simulink model "Closed_loop_Model_P_Controller"  (R2024b)
settings: Solver=VariableStepAuto  StartTime=0.0  StopTime=10.0  RelTol=1e-3
settings Model: Creator=Zohaib  LastModifiedBy=Zohaib

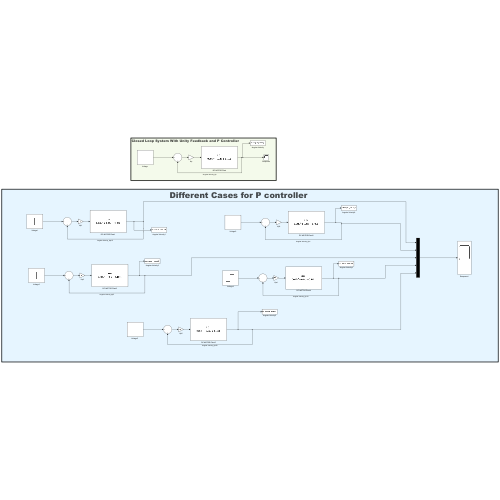
[thumbnail: Simulink's stored preview of the top-level diagram]
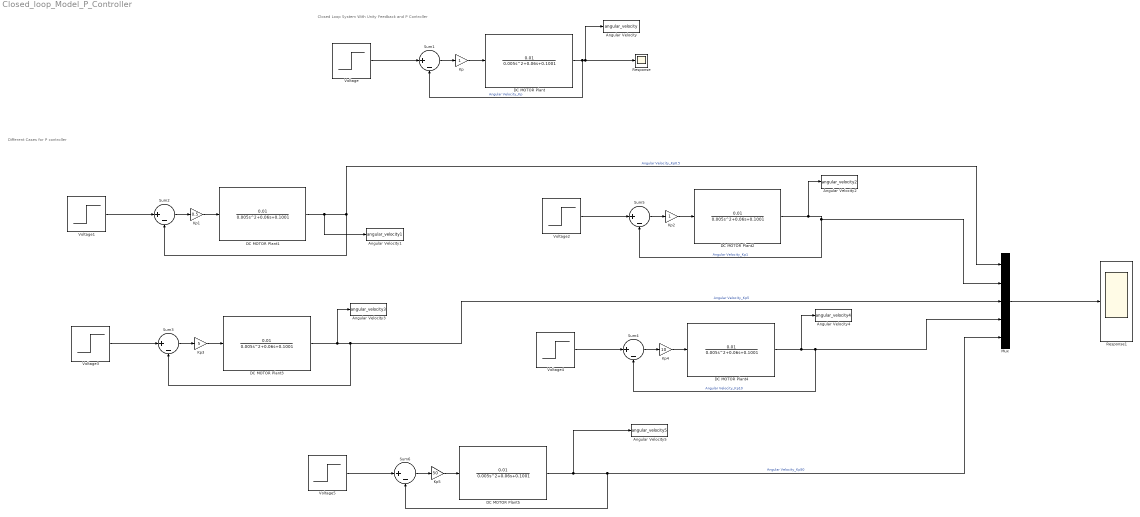
== system Closed_loop_Model_P_Controller ==
  note: Different Cases for P controller
  note: Closed Loop System With Unity Feedback and P Controller
  Angular Velocity : ToWorkspace  VariableName=angular_velocity  SaveFormat=Timeseries  SampleTime=-1
  Angular Velocity1 : ToWorkspace  VariableName=angular_velocity1  SaveFormat=Timeseries  SampleTime=-1
  Angular Velocity2 : ToWorkspace  VariableName=angular_velocity2  SaveFormat=Timeseries  SampleTime=-1
  Angular Velocity3 : ToWorkspace  VariableName=angular_velocity3  SaveFormat=Timeseries  SampleTime=-1
  Angular Velocity4 : ToWorkspace  VariableName=angular_velocity4  SaveFormat=Timeseries  SampleTime=-1
  Angular Velocity5 : ToWorkspace  VariableName=angular_velocity5  SaveFormat=Timeseries  SampleTime=-1
  DC MOTOR Plant{,1..5} (6 alike) : TransferFcn  Numerator=[0.01]  Denominator="[0.005  0.06  0.1001]"
  Kp : Gain
  Kp1 : Gain  Gain=0.5
  Kp2 : Gain
  Kp3 : Gain  Gain=5
  "Kp4 " : Gain  Gain=10
  Kp5 : Gain  Gain=50
  Mux : Mux  Inputs=5
  Response : Scope
  Response1 : Scope
  Sum{1..6} (6 alike) : Sum  Inputs=|+-
  "Voltage " : Step  SampleTime=0
  Voltage{1..4} (4 alike) : Step  SampleTime=0
  "Voltage5  " : Step  SampleTime=0
  wires:
  DC MOTOR Plant3/1 -> Angular Velocity3/1, Sum3/2, Mux/3  "Angular Velocity_Kp5"
  Voltage3/1 -> Sum3/1
  Sum3/1 -> Kp3/1
  Sum5/1 -> Kp2/1
  Kp2/1 -> DC MOTOR Plant2/1
  Voltage2/1 -> Sum5/1
  Sum4/1 -> "Kp4 "/1
  DC MOTOR Plant2/1 -> Angular Velocity2/1, Sum5/2, Mux/2  "Angular Velocity_Kp1"
  Sum1/1 -> Kp/1
  "Voltage "/1 -> Sum1/1
  DC MOTOR Plant/1 -> Response/1, Angular Velocity/1, Sum1/2  "Angular Velocity_Kp"
  Voltage4/1 -> Sum4/1
  Kp/1 -> DC MOTOR Plant/1
  Kp1/1 -> DC MOTOR Plant1/1
  "Kp4 "/1 -> DC MOTOR Plant4/1
  Voltage1/1 -> Sum2/1
  DC MOTOR Plant4/1 -> Angular Velocity4/1, Mux/4, Sum4/2  "Angular Velocity_Kp10"
  DC MOTOR Plant1/1 -> Sum2/2, Mux/1, Angular Velocity1/1  "Angular Velocity_Kp0.5"
  Sum2/1 -> Kp1/1
  Kp3/1 -> DC MOTOR Plant3/1
  DC MOTOR Plant5/1 -> Sum6/2, Mux/5, Angular Velocity5/1  "Angular Velocity_Kp50"
  "Voltage5  "/1 -> Sum6/1
  Sum6/1 -> Kp5/1
  Kp5/1 -> DC MOTOR Plant5/1
  Mux/1 -> Response1/1
